simulink model "week2_problem4"  (R2020b)
settings: Solver=VariableStepAuto  StartTime=0.0  StopTime=10.0  RelTol=1e-3
model workspace (MAT data in the model file):
  J = 3.2284e-06
  K = 0.0274
  Kd = 0.0508488040949
  Ki = 62.7263213782
  Kp = 4.02355957991
  L = 2.75e-06
  R = 4
  b = 3.5077e-06
settings Model: OrderedModelArguments=off  Creator=sai  LastModifiedBy=sai

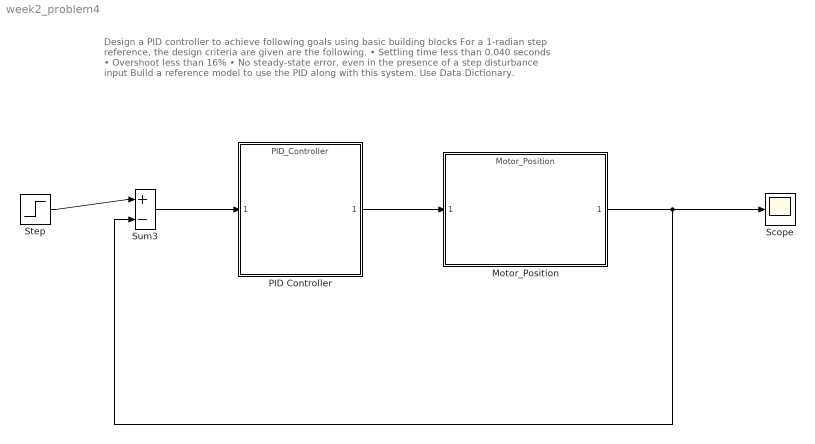
== system week2_problem4 ==
  note: Design a PID controller to achieve following goals using basic building blocks For a 1-radian step reference, the design criteria are given are the following. • Settling time less than 0.040 seconds • Overshoot less than 16% • No steady-state error, even in the presence of a step disturbance input Build a reference model to use the PID along with this system. Use Data Dictionary.
  Motor_Position : ModelReference  ModelNameDialog=Motor_Position  ModelReferenceVersion=1.1
  PID Controller : ModelReference  ModelNameDialog=PID_Controller  ModelReferenceVersion=1.2
  Scope : Scope
  Step : Step  SampleTime=0
  Sum3 : Sum  Inputs=|+-
  wires:
  Step/1 -> Sum3/1
  Motor_Position/1 -> Scope/1, Sum3/2
  Sum3/1 -> PID Controller/1
  PID Controller/1 -> Motor_Position/1
